simulink model "Nerthus_sim"  (R2021a)
settings: Solver=ode45  StartTime=0.0  StopTime=simtime  MaxStep=ts_max
values from neighbouring files (symbols this model uses):
  a_f = 1E-5*depl_fuel_temp_coef(depl_index)    [parameters.m]
  a_g = 1E-5*depl_grap_temp_coef(depl_index)    [parameters.m]
  A_s = 1.2245    [parameters.m]
  beta = depl_beta(depl_index,:)    [parameters.m]
  beta_t = sum(beta)    [parameters.m]
  Cp_1 = mean(interp1(Cal_temp1, Cal_Cp1, region_fdw))/1e3    [parameters.m]
  Cp_2 = mean(interp1(Cal_temp2, Cal_Cp2, region_sc))/1e3    [parameters.m]
  Cp_3 = mean(interp1(Cal_temp3, Cal_Cp3, region_s2))/1e3    [parameters.m]
  Cp_4 = mean(interp1(Cal_temp4, Cal_Cp4, region_s1))/1e3    [parameters.m]
  Cp_p = 0.00154912    [parameters.m]
  Cp_w = 456.056e-6    (= 0.000456056)    [parameters.m]
  D_it = 0.0141478    [parameters.m]
  D_ot = 0.015875    [parameters.m]
  DHRS_MODE = 1    [parameters.m]    (also in transients.m)
  DHRS_Power = P*(0.10)    (= 55.7)    [parameters.m]    (also in transients.m)
  DHRS_time = 20000000    [parameters.m]    (also in transients.m)
  DHRS_TIME_K = 10    [parameters.m]
  dHs_dPs = -0.042433622114357    (= -0.0424336221144)    [parameters.m]
  Epsilon = 1E-3    (= 0.001)    [parameters.m]
  Fiss_factor = 2.464783802008740e-03    (= 0.00246478380201)    [parameters.m]
  gamma0 = 9.635981959409105e-01    (= 0.963598195941)    [parameters.m]
  gamma1 = 3.560674858154914e-02    (= 0.0356067485815)    [parameters.m]
  gamma2 = 7.950554775404400e-04    (= 0.00079505547754)    [parameters.m]
  gamma_I = 5.1135e-2    (= 0.051135)    [parameters.m]
  gamma_Te = 6.1e-2    (= 0.061)    [parameters.m]
  gamma_Xe = 1.1628e-2    (= 0.011628)    [parameters.m]
  h_pw = h_s_shx    (= 0.00910134357894)    [parameters.m]
  H_s_table = zeros(m, n)    [parameters.m]
  h_wb = 13349.334646671E-6    (= 0.0133493346467)    [parameters.m]
  h_ws = 5732.378387768E-6    (= 0.00573237838777)    [parameters.m]
  h_wsc = 8385.005556375E-6    (= 0.00838500555638)    [parameters.m]
  hA_fg = 12.5325*SF_area_CORE    (= 12.5325)    [parameters.m]
  hA_p_phx1 = [UA_phx_nm,UA_phx_nm,UA_phx_nm,UA_phx_nm]    [parameters.m]
  hA_p_shx1 = [UA_shx_nm,UA_shx_nm,UA_shx_nm,UA_shx_nm]    [parameters.m]
  hA_s_phx1 = [UA_phx_nm,UA_phx_nm,UA_phx_nm,UA_phx_nm]    [parameters.m]
  hA_s_shx1 = [UA_shx_nm,UA_shx_nm,UA_shx_nm,UA_shx_nm]    [parameters.m]
  I_0 = ((gamma_I*Sig_f_msdr*phi_0) + (lam_Te*Te_0))/lam_I    (= 7.13664200441e+16)    [parameters.m]
  k_1 = 0.5    [parameters.m]
  K_1 = 11.632248097704855    (= 11.6322480977)    [parameters.m]
  k_2 = 0.5    [parameters.m]
  K_4 = b(1)    [parameters.m]
  K_5 = a(1)    [parameters.m]
  K_b = 12.834854076292217    (= 12.8348540763)    [parameters.m]
  k_f1 = k_f/nn_f    (= 0.465)    [parameters.m]
  k_f2 = k_f/nn_f    (= 0.465)    [parameters.m]
  k_g = 0.07    [parameters.m]
  K_pump = 10000000    [parameters.m]
  K_sc = -17.615718797133468    (= -17.6157187971)    [parameters.m]
  L = 8.5344*SF_length    (= 7.72866182253)    [parameters.m]
  L_b = 2.3645*SF_length    (= 2.14126603855)    [parameters.m]
  L_s = 4.723*SF_length    (= 4.27709854094)    [parameters.m]
  L_sc = 1.4469*SF_length    (= 1.31029724304)    [parameters.m]
  Lam = depl_Lam(depl_index)    [parameters.m]
  lam = [1.240E-02, 3.05E-02, 1.11E-01, 3.01E-01, 1.140E+00, 3.014E+00]    [parameters.m]
  lam_bubl = 2E-2    (= 0.02)    [parameters.m]
  lam_I = 2.875e-5    (= 2.875e-05)    [parameters.m]
  lam_Te = 3.65e-02    (= 0.0365)    [parameters.m]
  lam_Xe = 2.0916e-5    (= 2.0916e-05)    [parameters.m]
  lambda0 = 0.0945298    [parameters.m]
  lambda1 = 0.00441957    [parameters.m]
  lambda2 = 8.60979e-05    [parameters.m]
  m_f_t = mdot_fuel*(tau_core + tau_phx + tau_DHRS)    (= 116168.4)    [parameters.m]
  M_initial = L_b*rho_b*A_s + L_s*rho_s*A_s + L_sc*A_s*rho_sc    [parameters.m]
  M_stm = 0.018    [parameters.m]
  mcp_f1 = mn_f*scp_fuel    (= 62.07748875)    [parameters.m]
  mcp_f2 = mn_f*scp_fuel    (= 62.07748875)    [parameters.m]
  mcp_g1 = m_g*scp_graphite    (= 3731.2785)    [parameters.m]
  mcp_p_phx1 = scp_fuel*mp_phx1    [parameters.m]
  mcp_p_shx1 = scp_coolant*mp_shx1    [parameters.m]
  mcp_s_phx1 = scp_coolant*ms_phx1    [parameters.m]
  mcp_s_shx1 = scp_HITEC*ms_shx1    [parameters.m]
  mcp_t_phx1 = scp_tube*mt_phx1    [parameters.m]
  mcp_t_shx1 = scp_tube*mt_shx1    [parameters.m]
  mdot_coolant = 1543 + SF_fdw_PHX    (= 1543)    [parameters.m]
  mdot_HITEC = 3379 + SF_fdw_SHX    (= 3379)    [parameters.m]
  mn_f = (m_f/nn_f)    (= 31567.5)    [parameters.m]
  mn_piDHRS = mdot_fuel*tau_DHRS    (= 4209)    [parameters.m]
  mn_UHX = (tau_HITEC_UHX*mdot_HITEC)/n_UHX    (= 11263.3333333)    [parameters.m]
  mp_phx1 = [mp_phx_nm, mp_phx_nm, mp_phx_nm, mp_phx_nm]    [parameters.m]
  mp_shx1 = [mp_shx_nm, mp_shx_nm, mp_shx_nm, mp_shx_nm]    [parameters.m]
  ms_phx1 = [ms_phx_nm, ms_phx_nm, ms_phx_nm, ms_phx_nm]    [parameters.m]
  ms_shx1 = [ms_shx_nm, ms_shx_nm, ms_shx_nm, ms_shx_nm]    [parameters.m]
  N = 6546*SF_linear    (= 4861.496)    [parameters.m]
  n_frac0 = 1    [parameters.m]
  n_UHX = 3    [parameters.m]
  omega = 10.00000    (= 10)    [parameters.m]    (also in transients.m)
  P = 557    [parameters.m]    (also in transients.m)
  P_s = 12.5    [parameters.m]
  P_sat = 12.5    [parameters.m]
  P_sc = 12.5    [parameters.m]
  phi_0 = P/(3.04414e-17*1e6*Sig_f_msdr)    (= 3.1277117014e+14)    [parameters.m]
  Power_Bleed = P*(0.00)    (= 0)    [parameters.m]    (also in transients.m)
  pres_table = pres_inp    [parameters.m]
  R = 8.314462E-6    (= 8.314462e-06)    [parameters.m]
  rho_0 = beta_t - bterm    [parameters.m]
  rho_b = (XSteam('rho_pT', 125, 327.81) + XSteam('rho_pT', 125, 327.82))/2    [parameters.m]
  rho_p = rho_HITEC    (= 1680)    [parameters.m]
  rho_s = mean(interp1(Cal_temp_steam, Cal_rho3, region_steam))    [parameters.m]
  rho_sc = mean(interp1(Cal_temp2, Cal_rho2, region_sc))    [parameters.m]
  rho_w = 8425.712    [parameters.m]
  rhoXe_0 = (-sig_Xe / Sig_a) * (gamma_Te + gamma_I + gamma_Xe) * Sig_f_msdr * phi_0/(lam_Xe + sig_Xe * phi_0 + lam_bubl)    (= -0.000282704956487)    [parameters.m]
  scp_coolant = 8.83E-3    (= 0.00883)    [parameters.m]
  scp_fuel = 1.9665E-3    (= 0.0019665)    [parameters.m]
  scp_HITEC = 0.00154912    [parameters.m]
  Sig_f_msdr = U_den*U_sig    (= 0.058501076601)    [parameters.m]
  sig_Xe = 2.66449e-18    [parameters.m]
  sin_mag = 0    [parameters.m]    (also in transients.m)
  T0_f1 = Tf_in + (T0_f2-Tf_in)/2    (= 649.2)    [parameters.m]
  T0_f2 = 681.8    [parameters.m]
  T0_g1 = T0_f1 + (k_g*P/hA_fg)    (= 652.311111111)    [parameters.m]
  T0_p_phx1 = [663.1, 644.3, 630.3, 616.6]    [parameters.m]
  T0_p_shx1 = [641.8, 656.3, 621.4, 586.4]    [parameters.m]
  T0_s_phx1 = [595.1, 603.8, 615.6, 627.3]    [parameters.m]
  T0_s_shx1 = [598.2, 689.1, 651.4, 613.7]    [parameters.m]
  T0_t_phx1 = [639.3, 612.7]    [parameters.m]
  T0_t_shx1 = [646.6, 609.8]    [parameters.m]
  T_fw = 180.0    (= 180)    [parameters.m]
  T_p1 = 605.5    [parameters.m]
  T_p2 = 579.6    [parameters.m]
  T_p3 = 557.5    [parameters.m]
  ... (+40 more)
undefined symbols (not defined in the file or in its folder): C0, Cp_s, Cp_sc, ln, rho_f, scp_f, scp_s, vdot_f, vdot_s
libraries: pid_lib x1, simulink x1
(part 2 of 3)

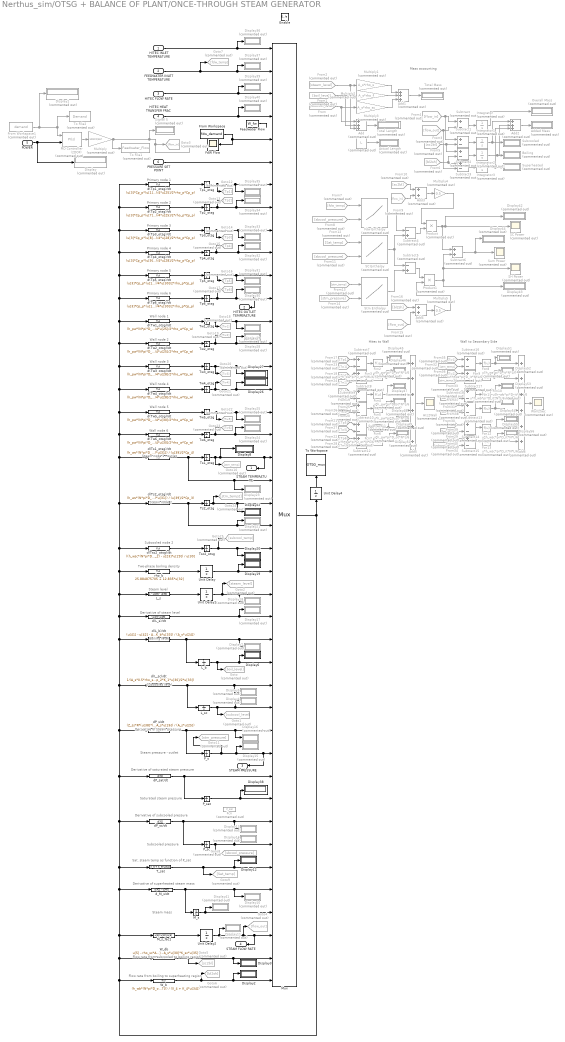
== system Nerthus_sim/OTSG + BALANCE OF PLANT/ONCE-THROUGH STEAM GENERATOR ==
  note: Wall to Secondary Side
  note: Hitec to Wall
  note: Mass accounting
  note: Primary node 1
  note: Primary node 2
  note: Primary node 3
  note: Primary node 4
  note: Primary node 5
  note: Primary node 6
  note: Wall node 1
  note: Wall node 2
  note: Wall node 3
  note: Wall node 4
  note: Wall node 5
  note: Wall node 6
  note: Steam node 1 - outlet
  note: Steam level
  note: Boiling level
  note: Subcooled level
  note: Derivative of saturated steam pressure
  note: Sat. steam temp as function of P_sat
  note: Saturated steam pressure
  note: Subcooled pressure
  note: Derivative of steam pressure
  note: Derivative of subcooled pressure
  note: Steam pressure - outlet
  note: Subcooled node 2
  note: Steam node 2
  note: Two-phase boiling density
  note: Derivative of superheated steam mass
  note: Steam mass
  note: Flow rate from subcooled to boiling region
  note: Flow rate from boiling to superheating region
  note: Derivative of steam level
  HITEC INLET TEMPERATURE : Inport
  FEEDWATER INLET TEMPERATURE : Inport  Port=2
  HITEC FLOW RATE : Inport  Port=3
  HITEC HEAT TRANSFER FRAC : Inport  Port=4
  POWER : Inport  Port=5
  PRESSURE SET POINT : Inport  Port=6
  Enable : EnablePort
  " " : Constant  Commented=on  Value=L
  "Actual Length " : Display  Commented=on
  Add : Sum  Commented=on  Inputs=+++
  Add1 : Sum  Commented=on  Inputs=+++
  Add2 : Sum  Commented=on  Inputs=+++
  Add3 : Sum  Commented=on
  Add4 : Sum  Commented=on
  Add5 : Sum  Commented=on  Inputs=++++++
  Add6 : Sum  Commented=on  Inputs=++++++
  Added Mass : Display  Commented=on
  Boiling : Display  Commented=on
  Display{,1,4..5,7,10..11,13..18,21,23..25,28..37,39..56} (45 alike) : Display  Commented=on
  Display{2..3,6,8,12,19..20,22,26..27,38} (11 alike) : Display
  Fcn : Fcn  Commented=on  Expr=P_sat
  Fcn10 : Fcn  Commented=on  Expr=u*h_wb*pi*D_it*N*L/6
  Fcn11 : Fcn  Commented=on  Expr=u*h_wb*pi*D_it*N*L/6
  Fcn12 : Fcn  Commented=on  Expr=u*h_wsc*pi*D_it*N*L/6
  Fcn13 : Fcn  Commented=on  Expr=u*h_wsc*pi*D_it*N*L/6
  Fcn{2..7} (6 alike) : Fcn  Commented=on  Expr=u*h_pw*pi*D_ot*N*L/6
  Fcn8 : Fcn  Commented=on  Expr=u*h_ws*pi*D_it*N*L/6
  Fcn9 : Fcn  Commented=on  Expr=u*h_ws*pi*D_it*N*L/6
  FdW Flow : Scope
  Fdw Enthalpy : Lookup_n-D  Commented=on  BreakpointsForDimension1=temp_table  BreakpointsForDimension2=pres_table  Table=H_s_table  DiagnosticForOutOfRangeInput=Warning  InternalRulePriority=Speed  RndMeth=Simplest  InputSameDT=on
      settings: InputPortMap=u0,u1
  Feedwater Flow : Constant  Value=W_fw
  From : From  Commented=on  GotoTag=subcool_level
  From Workspace : FromWorkspace  VariableName=fdw_demand
  From Workspace1 : FromWorkspace  Commented=on  VariableName=demand  SampleTime=1  Interpolate=off  OutputAfterFinalValue=Holding final value
  From1 : From  Commented=on  GotoTag=boil_level
  From10 : From  Commented=on  GotoTag=sc2bl
  From11 : From  Commented=on  GotoTag=sbcool_pressure
  From{12,29..31} (4 alike) : From  Commented=on  GotoTag=Sat_temp
  From13 : From  Commented=on  GotoTag=stm_temp
  From14 : From  Commented=on  GotoTag=stm_pressure
  From15 : From  Commented=on  GotoTag=flow_out
  From16 : From  Commented=on  GotoTag=bl2sh
  From17 : From  Commented=on  GotoTag=Tp1
  From18 : From  Commented=on  GotoTag=Tp2
  From19 : From  Commented=on  GotoTag=Tp3
  From2 : From  Commented=on  GotoTag=steam_level
  From20 : From  Commented=on  GotoTag=Tp4
  From21 : From  Commented=on  GotoTag=Tp5
  From22 : From  Commented=on  GotoTag=Tp6
  From23 : From  Commented=on  GotoTag=Tw1
  From24 : From  Commented=on  GotoTag=Tw2
  From25 : From  Commented=on  GotoTag=Tw3
  From26 : From  Commented=on  GotoTag=Tw4
  From27 : From  Commented=on  GotoTag=Tw5
  From28 : From  Commented=on  GotoTag=Tw6
  From3 : From  Commented=on  GotoTag=flow_out
  From32 : From  Commented=on  GotoTag=stm_temp
  From33 : From  Commented=on  GotoTag=stm_temp2
  From34 : From  Commented=on  GotoTag=subcool_temp
  From35 : From  Commented=on  GotoTag=Tw1
  From36 : From  Commented=on  GotoTag=Tw2
  From37 : From  Commented=on  GotoTag=Tw3
  From38 : From  Commented=on  GotoTag=Tw4
  From39 : From  Commented=on  GotoTag=Tw5
  From4 : From  Commented=on  GotoTag=flow_in
  From40 : From  Commented=on  GotoTag=Tw6
  From5 : From  Commented=on  GotoTag=sc2bl
  From6 : From  Commented=on  GotoTag=bl2sh
  From7 : From  Commented=on  GotoTag=fdw_temp
  From8 : From  Commented=on  GotoTag=sbcool_pressure
  From9 : From  Commented=on  GotoTag=flow_in
  Goto : Goto  Commented=on  GotoTag=boil_level
  Goto1 : Goto  Commented=on  GotoTag=subcool_level
  Goto10 : Goto  Commented=on  GotoTag=stm_temp
  Goto11 : Goto  Commented=on  GotoTag=stm_pressure
  Goto12 : Goto  Commented=on  GotoTag=Tp1
  Goto13 : Goto  Commented=on  GotoTag=Tp2
  Goto14 : Goto  Commented=on  GotoTag=Tp3
  Goto15 : Goto  Commented=on  GotoTag=Tp4
  Goto16 : Goto  Commented=on  GotoTag=Tp5
  Goto17 : Goto  Commented=on  GotoTag=Tp6
  Goto18 : Goto  Commented=on  GotoTag=Tw1
  Goto19 : Goto  Commented=on  GotoTag=Tw2
  Goto2 : Goto  Commented=on  GotoTag=steam_level
  Goto20 : Goto  Commented=on  GotoTag=Tw3
  Goto21 : Goto  Commented=on  GotoTag=Tw4
  Goto22 : Goto  Commented=on  GotoTag=Tw5
  Goto23 : Goto  Commented=on  GotoTag=Tw6
  Goto24 : Goto  Commented=on  GotoTag=stm_temp2
  Goto25 : Goto  Commented=on  GotoTag=subcool_temp
  Goto3 : Goto  Commented=on  GotoTag=flow_in
  Goto4 : Goto  Commented=on  GotoTag=flow_out
  Goto5 : Goto  Commented=on  GotoTag=sc2bl
  Goto6 : Goto  Commented=on  GotoTag=bl2sh
  Goto7 : Goto  Commented=on  GotoTag=fdw_temp
  Goto8 : Goto  Commented=on  GotoTag=sbcool_pressure
  Goto9 : Goto  Commented=on  GotoTag=Sat_temp
  Htc2Wall : Scope  Commented=on
  Integrator : Integrator  Commented=on  InitialCondition=M_initial
  Integrator1 : Integrator  Commented=on  InitialCondition=A_s*rho_sc*L_sc
  Integrator2 : Integrator  Commented=on  InitialCondition=A_s*rho_b*L_b
  Integrator3 : Integrator  Commented=on  InitialCondition=A_s*rho_s*L_s
  L_b : Integrator  InitialCondition=L_b  LimitOutput=on  LowerSaturationLimit=0.01
  L_s : Fcn  Expr=L - u[28] - u[30]
  L_sc : Integrator  InitialCondition=L_sc  LimitOutput=on  LowerSaturationLimit=0.01
  M_s : Integrator  InitialCondition=A_s*rho_s*L_s  LimitOutput=on  LowerSaturationLimit=1
  M_s_fac1 : Fcn  Expr=u[5]*u[32]/u[6]
  Multiply : Gain  Commented=on  Gain=1000*P/557
  Multiply1 : Gain  Commented=on  Gain=A_s*rho_s
  Multiply2 : Gain  Commented=on  Gain=A_s*rho_f
  Multiply3 : Gain  Commented=on  Gain=A_s*rho_sc
  Multiply4 : Gain  Commented=on  Gain=0.5
  Multiply5 : Gain  Commented=on  Gain=0.5
  Mux : Mux  Inputs=42
      settings: DisplayOption=signals
  Overall Mass : Display  Commented=on
  PID Controller (2DOF) : pid_lib/PID Controller (2DOF)  Commented=on  Controller=PI  Form=Parallel  TimeDomain=Continuous-time  UseExternalTs=off  SampleTime=-1  IntegratorMethod=Forward Euler  FilterMethod=Forward Euler  ControllerParametersSource=internal  P=0.003  I=0.001  D=-0.1  UseFilter=on  N=0.07  b=60  c=0.000385  TunerSelectOption=Transfer Function Based (PID Tuner App)  InitialConditionSource=internal  InitialConditionForIntegrator=0  InitialConditionForFilter=0  DifferentiatorICPrevScaledInput=0  ExternalReset=none  TrackingMode=off  Kt=1  LimitOutput=on  SatLimitsSource=internal  UpperSaturationLimit=2  LowerSaturationLimit=0.009  LinearizeAsGain=on  AntiWindupMode=none  Kb=1  POutMin=[]  POutMax=[]  IOutMin=[]  IOutMax=[]  DOutMin=[]  DOutMax=[]  NOutMin=[]  NOutMax=[]  bOutMin=[]  bOutMax=[]  cOutMin=[]  cOutMax=[]  SumOutMin=[]  SumOutMax=[]  SaturationOutMin=[]  SaturationOutMax=[]  PParamMin=[]  PParamMax=[]  IParamMin=[]  IParamMax=[]  DParamMin=[]  DParamMax=[]  NParamMin=[]  NParamMax=[]  bParamMin=[]  bParamMax=[]  cParamMin=[]  cParamMax=[]  KbParamMin=[]  KbParamMax=[]  KtParamMin=[]  KtParamMax=[]  KbOutMin=[]  KbOutMax=[]  KtOutMin=[]  KtOutMax=[]  IntegratorOutMin=[]  IntegratorOutMax=[]  FilterOutMin=[]  FilterOutMax=[]  SumI1OutMin=[]  SumI1OutMax=[]  SumI2OutMin=[]  SumI2OutMax=[]  SumI3OutMin=[]  SumI3OutMax=[]  SumI4OutMin=[]  SumI4OutMax=[]  SumDOutMin=[]  SumDOutMax=[]  Sum1OutMin=[]  Sum1OutMax=[]  Sum2OutMin=[]  Sum2OutMax=[]  Sum3OutMin=[]  Sum3OutMax=[]  DifferentiatorOutMin=[]  DifferentiatorOutMax=[]  FilterDiffOutCoefMin=[]  FilterDiffOutCoefMax=[]  ReciprocalOutMin=[]  ReciprocalOutMax=[]  SumDenOutMin=[]  SumDenOutMax=[]  SumNumOutMin=[]  SumNumOutMax=[]  DivideOutMin=[]  DivideOutMax=[]  UdiffTsProdOutMin=[]  UdiffTsProdOutMax=[]  NTsProdOutMin=[]  NTsProdOutMax=[]  UintegralTsProdOutMin=[]  UintegralTsProdOutMax=[]  UngainTsProdOutMin=[]  UngainTsProdOutMax=[]  IntegratorContinuousStateAttributes=''  IntegratorStateMustResolveToSignalObject=off  IntegratorRTWStateStorageClass=Auto  FilterContinuousStateAttributes=''  FilterStateMustResolveToSignalObject=off  FilterRTWStateStorageClass=Auto  ParallelPVariant=InternalParameters  IdealPVariant=Disabled  IVariant=InternalParameters  DVariant=Disabled  bVariant=InternalParameters  cVariant=Disabled  IntegratorVariant=Continuous  SatVariant=Enabled  AWVariant=Passthrough  PCopyVariant=Disabled  TRVariant=Disabled  FdbkBlocksVariant=Forward  IdealPFdbkVariant=Disabled  SatFdbkVariant=Disabled  DerivativeFilterVariant=Disabled  NVariant=Disabled  NCopyVariant=Disabled_SignalSpec  FilterICVariant=Disabled  IntegratorICVariant=InternalICs  ExternalResetVariant=Disabled  TRSumVariant=Passthrough  SumFdbkVariant=Disabled  SumVariant=Sum_PI  TsampFilterVariant=InternalTs  TsampNgainVariant=Passthrough  TsampIntegralVariant=Passthrough  ExternalSaturationOutDataTypeStr=Inherit: Same as second input
      settings: SourceProductBaseCode=SL
  P_s : Integrator  InitialCondition=P_s
  P_sat : Integrator  InitialCondition=P_sat
  P_sc : Integrator  InitialCondition=P_sc
  Product : Product  Commented=on
  Product1 : Product  Commented=on
  SC Enthalpy : Lookup_n-D  Commented=on  BreakpointsForDimension1=temp_table  BreakpointsForDimension2=pres_table  Table=H_s_table  DiagnosticForOutOfRangeInput=Warning  InternalRulePriority=Speed  RndMeth=Simplest  InputSameDT=on
      settings: InputPortMap=u0,u1
  SC Power : Scope  Commented=on
  SH Power : Scope  Commented=on
  Signal 5 : Display  Commented=on
  Stm Enthalpy : Lookup_n-D  Commented=on  BreakpointsForDimension1=temp_table  BreakpointsForDimension2=pres_table  Table=H_s_table  DiagnosticForOutOfRangeInput=Warning  InternalRulePriority=Speed  RndMeth=Simplest  InputSameDT=on
      settings: InputPortMap=u0,u1
  Subcooled : Display  Commented=on
  Subtract{,1..3,7..18} (16 alike) : Sum  Commented=on  Inputs=+-
  Subtract4 : Sum  Commented=on  Inputs=-+
  Subtract5 : Sum  Commented=on  Inputs=-+
  Subtract6 : Sum  Commented=on
  Sum Power : Scope  Commented=on
  Superheated : Display  Commented=on
  T_sat : Fcn  Expr=X_5 + K_5*u[34]
  To File1 : ToFile  Commented=on  Filename=Feedwater_Flow  MatrixName=Feedwater_Flow
  To File2 : ToFile  Commented=on  Filename=Demand  MatrixName=Demand
  To Workspace : ToWorkspace  VariableName=OTSG_mux  SaveFormat=Timeseries  SampleTime=-1
  Total Length : Display  Commented=on
  Total Mass : Display  Commented=on
  Tp1_otsg : Integrator  InitialCondition=T_p1
  Tp2_otsg : Integrator  InitialCondition=T_p2
  Tp3_otsg : Integrator  InitialCondition=T_p3
  Tp4_otsg : Integrator  InitialCondition=T_p4
  Tp5_otsg : Integrator  InitialCondition=T_p5
  Tp6_otsg : Integrator  InitialCondition=T_p6
  Ts1_otsg : Integrator  InitialCondition=T_s1
  Ts2_otsg : Integrator  InitialCondition=T_s2
  Tsc2_otsg : Integrator  InitialCondition=T_sc2
  Tw1_otsg : Integrator  InitialCondition=T_w1
  Tw2_otsg : Integrator  InitialCondition=T_w2
  Tw3_otsg : Integrator  InitialCondition=T_w3
  Tw4_otsg : Integrator  InitialCondition=T_w4
  Tw5_otsg : Integrator  InitialCondition=T_w5
  Tw6_otsg : Integrator  InitialCondition=T_w6
  Unit Delay : UnitDelay  InitialCondition=rho_b  SampleTime=-1  HasFrameUpgradeWarning=on
  Unit Delay1 : UnitDelay  InitialCondition=L_s  SampleTime=-1  HasFrameUpgradeWarning=on
  Unit Delay2 : UnitDelay  InitialCondition=W_fw  SampleTime=-1  HasFrameUpgradeWarning=on
  Unit Delay4 : UnitDelay  SampleTime=-1  HasFrameUpgradeWarning=on
  W_b : Fcn  Expr=(h_wb*(N*pi*D_ot*u[28])*(0.5*u[15] + 0.5*u[16] - u[37])) / (X_4 + K_4*u[34])
  W_db : Fcn  Expr=u[5] - rho_sc*A_s*u[29] - A_s*u[30]*K_sc*u[35]
  Wall2Sec : Scope  Commented=on
  d(L_b)/dt : Fcn  Expr=(u[41] - u[42] - A_s*u[28]*K_b*u[33]) / (A_s*u[24])
  d(L_s)/dt : Fcn  Expr=-u[27]-u[29]
  d(L_sc)/dt : Fcn  Expr=1/(A_s*0.5*rho_sc*Cp_2*(u[23] - u[37])) * (h_wsc*N*pi*D_ot*u[30]/2*(u[17] - u[37]) + Cp_2*(u[5]*u[23] - (u[5] + u[41])*0.5*u[37]) - A_s*u[30]/2*(K_sc*Cp_2*(u[23] - 2*u[37]) - 1)*u[35] - A_s*rho_sc*Cp_2*K_1*u[30]/2*u[33])
  d(Tp1_otsg)/dt : Fcn  Expr=(u[3]*Cp_p*(u[1] - u[7]) + h_pw*(N*pi*D_it*u[25]/2)*(u[13] - u[7])) / (N*pi*(D_it^2)/4*u[25]/2*rho_p*Cp_p)
  d(Tp2_otsg)/dt : Fcn  Expr=(u[3]*Cp_p*(u[7] - u[8]) + h_pw*(N*pi*D_it*u[25]/2)*(u[14] - u[8])) / (N*pi*(D_it^2)/4*u[25]/2*rho_p*Cp_p)
  d(Tp3_otsg)/dt : Fcn  Expr=(u[3]*Cp_p*(u[8] - u[9]) + h_pw*(N*pi*D_it*u[28]/2)*(u[15] - u[9])) / (N*pi*(D_it^2)/4*u[28]/2*rho_p*Cp_p)
  d(Tp4_otsg)/dt : Fcn  Expr=(u[3]*Cp_p*(u[9] - u[10]) + h_pw*(N*pi*D_it*u[28]/2)*(u[16] - u[10])) / (N*pi*(D_it^2)/4*u[28]/2*rho_p*Cp_p)
  d(Tp5_otsg)/dt : Fcn  Expr=(u[3]*Cp_p*(u[10] - u[11]) + h_pw*(N*pi*D_it*u[30]/2)*(u[17] - u[11])) / (N*pi*(D_it^2)/4*u[30]/2*rho_p*Cp_p)
  d(Tp6_otsg)/dt : Fcn  Expr=(u[3]*Cp_p*(u[11] - u[12]) + h_pw*(N*pi*D_it*u[30]/2)*(u[18] - u[12])) / (N*pi*(D_it^2)/4*u[30]/2*rho_p*Cp_p)
  d(Ts1_otsg)/dt : Fcn  Expr=(h_ws*(N*pi*D_ot*u[25]/2)*(u[13] - u[19]) + u[40]*Cp_4*(u[21] - u[19]) + Cp_4*(u[21] - u[19])*u[38]/2 + (A_s*u[25]/2 - u[39]/2*dHs_dPs)*u[31]) / (u[39]/2*Cp_4)
  d(Ts2_otsg)/dt : Fcn  Expr=(h_ws*(N*pi*D_ot*u[25]/2)*(u[14] - u[21]) + u[42]*Cp_3*(u[37] - u[21]) + (A_s*u[25]/2 - u[39]/2*dHs_dPs)*u[31]) / (u[39]/2*Cp_3)
  d(Tsc2_otsg)/dt : Fcn  Expr=((h_wsc*(N*pi*D_ot*u[30]/2)*(u[18] - u[23]) + (Cp_1*u[5]*u[2]) - Cp_2*((u[5] + u[41])*0.5*u[23]) + A_s*u[30]/2*u[35]) * 2/(A_s*rho_sc*Cp_2) - u[23]*u[29]) / u[30]
  d(Tw1_otsg)/dt : Fcn  Expr=(h_pw*(N*pi*D_it*u[25]/2)*(u[7] - u[13]) + h_ws*(N*pi*D_ot*u[25]/2)*(u[19] - u[13])) / (N*pi*(D_ot^2 - D_it^2)/4*u[25]/2*rho_w*Cp_w)
  d(Tw2_otsg)/dt : Fcn  Expr=(h_pw*(N*pi*D_it*u[25]/2)*(u[8] - u[14]) + h_ws*(N*pi*D_ot*u[25]/2)*(u[21] - u[14])) / (N*pi*(D_ot^2 - D_it^2)/4*u[25]/2*rho_w*Cp_w)
  d(Tw3_otsg)/dt : Fcn  Expr=(h_pw*(N*pi*D_it*u[28]/2)*(u[9] - u[15]) + h_wb*(N*pi*D_ot*u[28]/2)*(u[37] - u[15])) / (N*pi*(D_ot^2 - D_it^2)/4*u[28]/2*rho_w*Cp_w)
  d(Tw4_otsg)/dt : Fcn  Expr=(h_pw*(N*pi*D_it*u[28]/2)*(u[10] - u[16]) + h_wb*(N*pi*D_ot*u[28]/2)*(u[37] - u[16])) / (N*pi*(D_ot^2 - D_it^2)/4*u[28]/2*rho_w*Cp_w)
  d(Tw5_otsg)/dt : Fcn  Expr=(h_pw*(N*pi*D_it*u[30]/2)*(u[11] - u[17]) + h_wsc*(N*pi*D_ot*u[30]/2)*(u[37] - u[17])) / (N*pi*(D_ot^2 - D_it^2)/4*u[30]/2*rho_w*Cp_w)
  d(Tw6_otsg)/dt : Fcn  Expr=(h_pw*(N*pi*D_it*u[30]/2)*(u[12] - u[18]) + h_wsc*(N*pi*D_ot*u[30]/2)*(u[23] - u[18])) / (N*pi*(D_ot^2 - D_it^2)/4*u[30]/2*rho_w*Cp_w)
  dP_s/dt : Fcn  Expr=(Z_ss*R*(u[38]*(u[19] + u[21]) + u[39]*(u[20] + u[22]))/(2*M_stm) - u[32]*A_s*u[26]) / (A_s*u[25])
  dP_sat/dt : Fcn  Expr=u[31]
  dP_sc/dt : Fcn  Expr=u[31]
  d_M_s/dt : Fcn  Expr=u[42] - u[40]
  rho_b : Fcn  Expr=25.884875705 + 12.835*u[32]
  STEAM TEMPERATURE : Outport  VectorParamsAs1DForOutWhenUnconnected=off
  HITEC OUTLET TEMPERATURE : Outport  Port=2  VectorParamsAs1DForOutWhenUnconnected=off
  STEAM PRESSURE : Outport  Port=3  VectorParamsAs1DForOutWhenUnconnected=off
  STEAM FLOW RATE : Outport  Port=4  VectorParamsAs1DForOutWhenUnconnected=off
  wires:
  d(Tp1_otsg)/dt/1 -> Tp1_otsg/1
  HITEC INLET TEMPERATURE/1 -> Display36/1, Mux/1
  HITEC FLOW RATE/1 -> Display39/1, Mux/3
  HITEC HEAT TRANSFER FRAC/1 -> Display40/1, Mux/4
  PRESSURE SET POINT/1 -> Mux/6
  Tp1_otsg/1 -> Goto12/1, Display35/1, Mux/7
  Tp2_otsg/1 -> Goto13/1, Display34/1, Mux/8
  d(Tp2_otsg)/dt/1 -> Tp2_otsg/1
  Tp3_otsg/1 -> Goto14/1, Display33/1, Mux/9
  d(Tp3_otsg)/dt/1 -> Tp3_otsg/1
  Tp4_otsg/1 -> Goto15/1, Display32/1, Mux/10
  d(Tp4_otsg)/dt/1 -> Tp4_otsg/1
  Tp5_otsg/1 -> Goto16/1, Display31/1, Mux/11
  d(Tp5_otsg)/dt/1 -> Tp5_otsg/1
  d(Tp6_otsg)/dt/1 -> Tp6_otsg/1
  Tp6_otsg/1 -> Goto17/1, Display30/1, HITEC OUTLET TEMPERATURE/1, Mux/12
  d(Tw1_otsg)/dt/1 -> Tw1_otsg/1
  d(Tw2_otsg)/dt/1 -> Tw2_otsg/1
  Tw3_otsg/1 -> Goto20/1, Display27/1, Mux/15
  d(Tw3_otsg)/dt/1 -> Tw3_otsg/1
  d(Tw4_otsg)/dt/1 -> Tw4_otsg/1
  Tw4_otsg/1 -> Goto21/1, Display26/1, Mux/16
  Tw5_otsg/1 -> Goto22/1, Display25/1, Mux/17
  d(Tw5_otsg)/dt/1 -> Tw5_otsg/1
  d(Tw6_otsg)/dt/1 -> Tw6_otsg/1
  Tw6_otsg/1 -> Goto23/1, Display24/1, Mux/18
  L_sc/1 -> Goto1/1, Display4/1, Mux/30
  L_s/1 -> Unit Delay1/1
  L_b/1 -> Goto/1, Display6/1, Mux/28
  P_sat/1 -> Display38/1, Mux/34
  Tsc2_otsg/1 -> Goto25/1, Display20/1, Mux/23
  d(Tsc2_otsg)/dt/1 -> Tsc2_otsg/1
  Ts2_otsg/1 -> Goto24/1, Display22/1, Mux/21
  rho_b/1 -> Unit Delay/1
  Unit Delay/1 -> Display19/1, Mux/24
  d(Ts1_otsg)/dt/1 -> Display23/1, Mux/20, Ts1_otsg/1
  d(Ts2_otsg)/dt/1 -> Display21/1, Mux/22, Ts2_otsg/1
  dP_s/dt/1 -> Display16/1, Mux/31, P_s/1
  d(L_b)/dt/1 -> Display7/1, Mux/27, L_b/1
  d(L_s)/dt/1 -> Display17/1, Mux/26
  d(L_sc)/dt/1 -> Display5/1, Mux/29, L_sc/1
  dP_sat/dt/1 -> Mux/33, P_sat/1
  dP_sc/dt/1 -> Display13/1, Mux/35, P_sc/1
  Unit Delay1/1 -> Goto2/1, Display18/1, Mux/25
  T_sat/1 -> Goto9/1, Display12/1, Mux/37
  M_s_fac1/1 -> Unit Delay2/1
  d_M_s/dt/1 -> Display10/1, Mux/38, M_s/1
  Unit Delay4/1 -> To Workspace/1
  Tw1_otsg/1 -> Goto18/1, Display29/1, Mux/13
  From Workspace1/1 -> PID Controller (2DOF)/1, To File2/1, Display1/1
  Ts1_otsg/1 -> Goto10/1, STEAM TEMPERATURE/1, Mux/19, Display8/1
  POWER/1 -> PID Controller (2DOF)/2, Display/1
  Tw2_otsg/1 -> Goto19/1, Display28/1, Mux/14
  P_s/1 -> Goto11/1, Display15/1, Mux/32, STEAM PRESSURE/1
  Unit Delay2/1 -> Goto4/1, STEAM FLOW RATE/1, Mux/40, Display11/1
  P_sc/1 -> Goto8/1, Display14/1, Mux/36
  FEEDWATER INLET TEMPERATURE/1 -> Goto7/1, Display37/1, Mux/2
  PID Controller (2DOF)/1 -> Multiply/1
  From/1 -> Add/1, Multiply3/1
  From1/1 -> Multiply2/1, Add/2
  From2/1 -> Add/3, Multiply1/1
  Add/1 -> Total Length/1
  " "/1 -> "Actual Length "/1
  Multiply3/1 -> Add1/3
  Multiply2/1 -> Add1/2
  Multiply1/1 -> Add1/1
  Add1/1 -> Total Mass/1
  From4/1 -> Subtract1/1, Subtract/1
  From3/1 -> Subtract3/2, Subtract/2
  Subtract/1 -> Integrator/1
  M_s/1 -> Display41/1, Mux/39
  From5/1 -> Subtract2/1, Subtract1/2
  Subtract1/1 -> Integrator1/1
  Integrator1/1 -> Add2/1, Subcooled/1
  From6/1 -> Subtract2/2, Subtract3/1
  Integrator2/1 -> Add2/2, Boiling/1
  Subtract2/1 -> Integrator2/1
  Integrator3/1 -> Add2/3, Superheated/1
  Subtract3/1 -> Integrator3/1
  Add2/1 -> Added Mass/1
  Integrator/1 -> Overall Mass/1
  From7/1 -> Fdw Enthalpy/1
  From8/1 -> Fdw Enthalpy/2
  Fdw Enthalpy/1 -> Subtract4/1
  From9/1 -> Add3/2
  Product/1 -> Subtract6/1, Display42/1, SC Power/1
  From10/1 -> Add3/1
  Add3/1 -> Multiply4/1
  From11/1 -> SC Enthalpy/2
  From12/1 -> SC Enthalpy/1
  SC Enthalpy/1 -> Subtract4/2, Subtract5/1
  Multiply4/1 -> Product/1
  Subtract4/1 -> Product/2
  Stm Enthalpy/1 -> Subtract5/2
  From13/1 -> Stm Enthalpy/1
  From14/1 -> Stm Enthalpy/2
  From16/1 -> Add4/1
  Add4/1 -> Multiply5/1
  Multiply5/1 -> Product1/2
  From15/1 -> Add4/2
  Subtract5/1 -> Product1/1
  Product1/1 -> Subtract6/2, SH Power/1, Display43/1
  Subtract6/1 -> Display44/1, Sum Power/1
  From17/1 -> Subtract7/1
  From23/1 -> Subtract7/2
  From18/1 -> Subtract8/1
  From24/1 -> Subtract8/2
  From19/1 -> Subtract9/1
  From25/1 -> Subtract9/2
  From26/1 -> Subtract10/2
  From20/1 -> Subtract10/1
  From21/1 -> Subtract11/1
  From27/1 -> Subtract11/2
  From22/1 -> Subtract12/1
  From28/1 -> Subtract12/2
  Subtract7/1 -> Fcn2/1
  Subtract8/1 -> Fcn3/1
  Subtract9/1 -> Fcn4/1
  Subtract10/1 -> Fcn5/1
  Subtract11/1 -> Fcn6/1
  Subtract12/1 -> Fcn7/1
  Fcn2/1 -> Display45/1, Add5/1
  Fcn3/1 -> Display46/1, Add5/2
  Fcn4/1 -> Display47/1, Add5/3
  Fcn5/1 -> Display48/1, Add5/4
  Fcn6/1 -> Display49/1, Add5/5
  Fcn7/1 -> Display50/1, Add5/6
  Add5/1 -> Htc2Wall/1
  Fcn9/1 -> Display52/1, Add6/2
  Add6/1 -> Wall2Sec/1
  Fcn10/1 -> Display53/1, Add6/3
  Fcn12/1 -> Display55/1, Add6/5
  Fcn13/1 -> Display56/1, Add6/6
  Fcn11/1 -> Display54/1, Add6/4
  Subtract16/1 -> Fcn8/1
  From36/1 -> Subtract17/1
  Fcn8/1 -> Display51/1, Add6/1
  Subtract13/1 -> Fcn11/1
  Subtract15/1 -> Fcn13/1
  From35/1 -> Subtract16/1
  Subtract17/1 -> Fcn9/1
  Subtract18/1 -> Fcn10/1
  Subtract14/1 -> Fcn12/1
  From40/1 -> Subtract15/1
  From39/1 -> Subtract14/1
  From37/1 -> Subtract18/1
  From38/1 -> Subtract13/1
  From29/1 -> Subtract14/2
  From30/1 -> Subtract13/2
  From31/1 -> Subtract18/2
  From32/1 -> Subtract16/2
  From33/1 -> Subtract17/2
  From34/1 -> Subtract15/2
  Multiply/1 -> To File1/1, Signal 5/1, Goto3/1
  Feedwater Flow/1 -> ?
  From Workspace/1 -> FdW Flow/1, Mux/5
  Mux/1 -> W_b/1, W_db/1, d_M_s/dt/1, T_sat/1, dP_sc/dt/1, dP_sat/dt/1, dP_s/dt/1, d(L_sc)/dt/1, d(L_b)/dt/1, d(L_s)/dt/1, L_s/1, rho_b/1, d(Tsc2_otsg)/dt/1, d(Ts2_otsg)/dt/1, d(Ts1_otsg)/dt/1, d(Tw6_otsg)/dt/1, d(Tw5_otsg)/dt/1, d(Tw4_otsg)/dt/1, d(Tw3_otsg)/dt/1, d(Tw2_otsg)/dt/1, d(Tw1_otsg)/dt/1, d(Tp6_otsg)/dt/1, d(Tp5_otsg)/dt/1, d(Tp4_otsg)/dt/1, d(Tp3_otsg)/dt/1, d(Tp2_otsg)/dt/1, d(Tp1_otsg)/dt/1, M_s_fac1/1, Unit Delay4/1
  W_b/1 -> Display2/1, Mux/42, Goto6/1
  W_db/1 -> Display3/1, Mux/41, Goto5/1

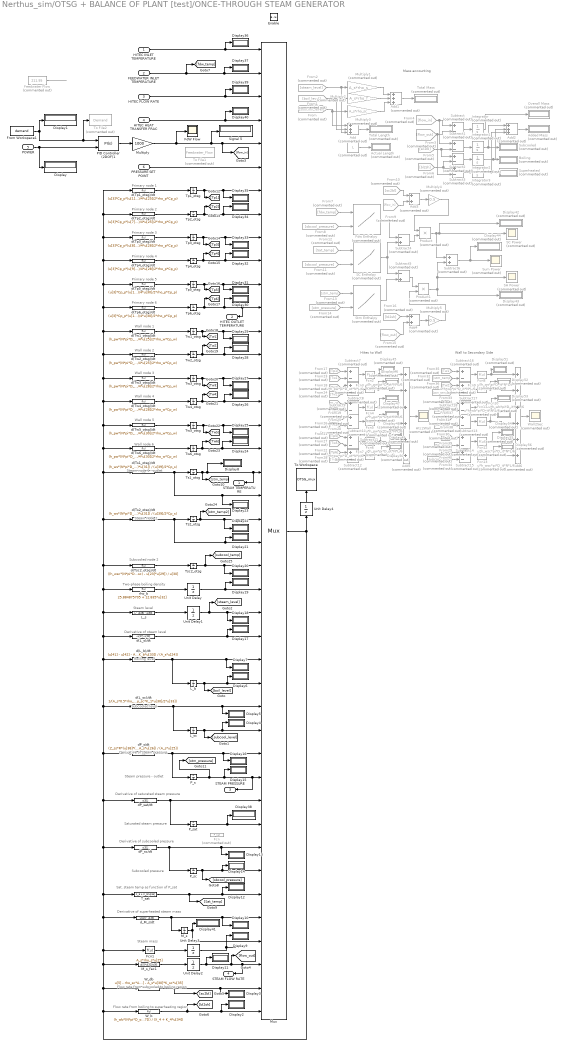
== system Nerthus_sim/OTSG + BALANCE OF PLANT [test]/ONCE-THROUGH STEAM GENERATOR ==
  note: Wall to Secondary Side
  note: Hitec to Wall
  note: Mass accounting
  note: Primary node 1
  note: Primary node 2
  note: Primary node 3
  note: Primary node 4
  note: Primary node 5
  note: Primary node 6
  note: Wall node 1
  note: Wall node 2
  note: Wall node 3
  note: Wall node 4
  note: Wall node 5
  note: Wall node 6
  note: Steam node 1 - outlet
  note: Steam level
  note: Boiling level
  note: Subcooled level
  note: Derivative of saturated steam pressure
  note: Sat. steam temp as function of P_sat
  note: Saturated steam pressure
  note: Subcooled pressure
  note: Derivative of steam pressure
  note: Derivative of subcooled pressure
  note: Steam pressure - outlet
  note: Subcooled node 2
  note: Steam node 2
  note: Two-phase boiling density
  note: Derivative of superheated steam mass
  note: Steam mass
  note: Flow rate from subcooled to boiling region
  note: Flow rate from boiling to superheating region
  note: Derivative of steam level
  HITEC INLET TEMPERATURE : Inport
  FEEDWATER INLET TEMPERATURE : Inport  Port=2
  HITEC FLOW RATE : Inport  Port=3
  HITEC HEAT TRANSFER FRAC : Inport  Port=4
  POWER : Inport  Port=5
  PRESSURE SET POINT : Inport  Port=6
  Enable : EnablePort
  " " : Constant  Commented=on  Value=L
  "Actual Length " : Display  Commented=on
  Add : Sum  Commented=on  Inputs=+++
  Add1 : Sum  Commented=on  Inputs=+++
  Add2 : Sum  Commented=on  Inputs=+++
  Add3 : Sum  Commented=on
  Add4 : Sum  Commented=on
  Add5 : Sum  Commented=on  Inputs=++++++
  Add6 : Sum  Commented=on  Inputs=++++++
  Added Mass : Display  Commented=on
  Boiling : Display  Commented=on
  Display{,1..41} (42 alike) : Display
  Display{42..56} (15 alike) : Display  Commented=on
  Fcn : Fcn  Commented=on  Expr=P_sat
  Fcn1 : Fcn  Expr=A_s*rho_s*u[25]
  Fcn10 : Fcn  Commented=on  Expr=u*h_wb*pi*D_it*N*L/6
  Fcn11 : Fcn  Commented=on  Expr=u*h_wb*pi*D_it*N*L/6
  Fcn12 : Fcn  Commented=on  Expr=u*h_wsc*pi*D_it*N*L/6
  Fcn13 : Fcn  Commented=on  Expr=u*h_wsc*pi*D_it*N*L/6
  Fcn{2..7} (6 alike) : Fcn  Commented=on  Expr=u*h_pw*pi*D_ot*N*L/6
  Fcn8 : Fcn  Commented=on  Expr=u*h_ws*pi*D_it*N*L/6
  Fcn9 : Fcn  Commented=on  Expr=u*h_ws*pi*D_it*N*L/6
  FdW Flow : Scope
  Fdw Enthalpy : Lookup_n-D  Commented=on  BreakpointsForDimension1=temp_table  BreakpointsForDimension2=pres_table  Table=H_s_table  DiagnosticForOutOfRangeInput=Warning  InternalRulePriority=Speed  RndMeth=Simplest  InputSameDT=on
      settings: InputPortMap=u0,u1
  "Feedwater Flow " : Constant  Commented=on  Value=211.95
  From : From  Commented=on  GotoTag=subcool_level
  From Workspace1 : FromWorkspace  VariableName=demand  SampleTime=1  Interpolate=off  OutputAfterFinalValue=Holding final value
  From1 : From  Commented=on  GotoTag=boil_level
  From10 : From  Commented=on  GotoTag=sc2bl
  From11 : From  Commented=on  GotoTag=sbcool_pressure
  From{12,29..31} (4 alike) : From  Commented=on  GotoTag=Sat_temp
  From13 : From  Commented=on  GotoTag=stm_temp
  From14 : From  Commented=on  GotoTag=stm_pressure
  From15 : From  Commented=on  GotoTag=flow_out
  From16 : From  Commented=on  GotoTag=bl2sh
  From17 : From  Commented=on  GotoTag=Tp1
  From18 : From  Commented=on  GotoTag=Tp2
  From19 : From  Commented=on  GotoTag=Tp3
  From2 : From  Commented=on  GotoTag=steam_level
  From20 : From  Commented=on  GotoTag=Tp4
  From21 : From  Commented=on  GotoTag=Tp5
  From22 : From  Commented=on  GotoTag=Tp6
  From23 : From  Commented=on  GotoTag=Tw1
  From24 : From  Commented=on  GotoTag=Tw2
  From25 : From  Commented=on  GotoTag=Tw3
  From26 : From  Commented=on  GotoTag=Tw4
  From27 : From  Commented=on  GotoTag=Tw5
  From28 : From  Commented=on  GotoTag=Tw6
  From3 : From  Commented=on  GotoTag=flow_out
  From32 : From  Commented=on  GotoTag=stm_temp
  From33 : From  Commented=on  GotoTag=stm_temp2
  From34 : From  Commented=on  GotoTag=subcool_temp
  From35 : From  Commented=on  GotoTag=Tw1
  From36 : From  Commented=on  GotoTag=Tw2
  From37 : From  Commented=on  GotoTag=Tw3
  From38 : From  Commented=on  GotoTag=Tw4
  From39 : From  Commented=on  GotoTag=Tw5
  From4 : From  Commented=on  GotoTag=flow_in
  From40 : From  Commented=on  GotoTag=Tw6
  From5 : From  Commented=on  GotoTag=sc2bl
  From6 : From  Commented=on  GotoTag=bl2sh
  From7 : From  Commented=on  GotoTag=fdw_temp
  From8 : From  Commented=on  GotoTag=sbcool_pressure
  From9 : From  Commented=on  GotoTag=flow_in
  Htc2Wall : Scope  Commented=on
  Integrator : Integrator  Commented=on  InitialCondition=M_initial
  Integrator1 : Integrator  Commented=on  InitialCondition=A_s*rho_sc*L_sc
  Integrator2 : Integrator  Commented=on  InitialCondition=A_s*rho_b*L_b
  Integrator3 : Integrator  Commented=on  InitialCondition=A_s*rho_s*L_s
  L_b : Integrator  InitialCondition=L_b
  L_s : Fcn  Expr=L - u[28] - u[30]
  L_sc : Integrator  InitialCondition=L_sc
  M_s : Integrator  InitialCondition=A_s*rho_s*L_s
  M_s_fac1 : Fcn  Expr=u[5]*u[32]/u[6]
  Multiply : Gain  Gain=1000
  Multiply1 : Gain  Commented=on  Gain=A_s*rho_s
  Multiply2 : Gain  Commented=on  Gain=A_s*rho_f
  Multiply3 : Gain  Commented=on  Gain=A_s*rho_sc
  Multiply4 : Gain  Commented=on  Gain=0.5
  Multiply5 : Gain  Commented=on  Gain=0.5
  Mux : Mux  Inputs=42
      settings: DisplayOption=signals
  Overall Mass : Display  Commented=on
  PID Controller (2DOF)1 : simulink/Continuous/PID Controller (2DOF)  Controller=PI  Form=Parallel  TimeDomain=Continuous-time  SampleTime=-1  IntegratorMethod=Forward Euler  FilterMethod=Forward Euler  ControllerParametersSource=internal  P=0.003  I=0.001  D=-0.1  UseFilter=on  N=0.07  b=60  c=0.000385  TunerSelectOption=Transfer Function Based (PID Tuner App)  InitialConditionSource=internal  InitialConditionForIntegrator=0  InitialConditionForFilter=0  DifferentiatorICPrevScaledInput=0  ExternalReset=none  TrackingMode=off  Kt=1  LimitOutput=on  UpperSaturationLimit=2  LowerSaturationLimit=0.001  LinearizeAsGain=on  AntiWindupMode=none  Kb=1  POutMin=[]  POutMax=[]  IOutMin=[]  IOutMax=[]  DOutMin=[]  DOutMax=[]  NOutMin=[]  NOutMax=[]  bOutMin=[]  bOutMax=[]  cOutMin=[]  cOutMax=[]  SumOutMin=[]  SumOutMax=[]  SaturationOutMin=[]  SaturationOutMax=[]  PParamMin=[]  PParamMax=[]  IParamMin=[]  IParamMax=[]  DParamMin=[]  DParamMax=[]  NParamMin=[]  NParamMax=[]  bParamMin=[]  bParamMax=[]  cParamMin=[]  cParamMax=[]  KbParamMin=[]  KbParamMax=[]  KtParamMin=[]  KtParamMax=[]  KbOutMin=[]  KbOutMax=[]  KtOutMin=[]  KtOutMax=[]  IntegratorOutMin=[]  IntegratorOutMax=[]  FilterOutMin=[]  FilterOutMax=[]  SumI1OutMin=[]  SumI1OutMax=[]  SumI2OutMin=[]  SumI2OutMax=[]  SumI3OutMin=[]  SumI3OutMax=[]  SumI4OutMin=[]  SumI4OutMax=[]  SumDOutMin=[]  SumDOutMax=[]  Sum1OutMin=[]  Sum1OutMax=[]  Sum2OutMin=[]  Sum2OutMax=[]  Sum3OutMin=[]  Sum3OutMax=[]  DifferentiatorOutMin=[]  DifferentiatorOutMax=[]  FilterDiffOutCoefMin=[]  FilterDiffOutCoefMax=[]  ReciprocalOutMin=[]  ReciprocalOutMax=[]  SumDenOutMin=[]  SumDenOutMax=[]  SumNumOutMin=[]  SumNumOutMax=[]  DivideOutMin=[]  DivideOutMax=[]  IntegratorContinuousStateAttributes=''  IntegratorStateMustResolveToSignalObject=off  IntegratorRTWStateStorageClass=Auto  FilterContinuousStateAttributes=''  FilterStateMustResolveToSignalObject=off  FilterRTWStateStorageClass=Auto  ParallelPVariant=InternalParameters  IdealPVariant=Disabled  IVariant=InternalParameters  DVariant=Disabled  bVariant=InternalParameters  cVariant=Disabled  IntegratorVariant=Continuous  SatVariant=Enabled  AWVariant=Passthrough  PCopyVariant=Disabled  TRVariant=Disabled  FdbkBlocksVariant=Forward  IdealPFdbkVariant=Disabled  SatFdbkVariant=Disabled  DerivativeFilterVariant=Disabled  NVariant=Disabled  NCopyVariant=Disabled_SignalSpec  FilterICVariant=Disabled  IntegratorICVariant=InternalICs  ExternalResetVariant=Disabled  TRSumVariant=Passthrough  SumFdbkVariant=Disabled  SumVariant=Sum_PI
  P_s : Integrator  InitialCondition=P_s
  P_sat : Integrator  InitialCondition=P_sat
  P_sc : Integrator  InitialCondition=P_sc
  Product : Product  Commented=on
  Product1 : Product  Commented=on
  SC Enthalpy : Lookup_n-D  Commented=on  BreakpointsForDimension1=temp_table  BreakpointsForDimension2=pres_table  Table=H_s_table  DiagnosticForOutOfRangeInput=Warning  InternalRulePriority=Speed  RndMeth=Simplest  InputSameDT=on
      settings: InputPortMap=u0,u1
  SC Power : Scope  Commented=on
  SH Power : Scope  Commented=on
  Signal 5 : Display
  Stm Enthalpy : Lookup_n-D  Commented=on  BreakpointsForDimension1=temp_table  BreakpointsForDimension2=pres_table  Table=H_s_table  DiagnosticForOutOfRangeInput=Warning  InternalRulePriority=Speed  RndMeth=Simplest  InputSameDT=on
      settings: InputPortMap=u0,u1
  Subcooled : Display  Commented=on
  Subtract{,1..3,7..18} (16 alike) : Sum  Commented=on  Inputs=+-
  Subtract4 : Sum  Commented=on  Inputs=-+
  Subtract5 : Sum  Commented=on  Inputs=-+
  Subtract6 : Sum  Commented=on
  Sum Power : Scope  Commented=on
  Superheated : Display  Commented=on
  T_sat : Fcn  Expr=X_5 + K_5*u[34]
  To File1 : ToFile  Commented=on  Filename=Feedwater_Flow  MatrixName=Feedwater_Flow
  To File2 : ToFile  Commented=on  Filename=Demand  MatrixName=Demand
  To Workspace : ToWorkspace  VariableName=OTSG_mux  SaveFormat=Timeseries  SampleTime=-1
  Total Length : Display  Commented=on
  Total Mass : Display  Commented=on
  Tp1_otsg : Integrator  InitialCondition=T_p1
  Tp2_otsg : Integrator  InitialCondition=T_p2
  Tp3_otsg : Integrator  InitialCondition=T_p3
  Tp4_otsg : Integrator  InitialCondition=T_p4
  Tp5_otsg : Integrator  InitialCondition=T_p5
  Tp6_otsg : Integrator  InitialCondition=T_p6
  Ts1_otsg : Integrator  InitialCondition=T_s1
  Ts2_otsg : Integrator  InitialCondition=T_s2
  Tsc2_otsg : Integrator  InitialCondition=T_sc2
  Tw1_otsg : Integrator  InitialCondition=T_w1
  Tw2_otsg : Integrator  InitialCondition=T_w2
  Tw3_otsg : Integrator  InitialCondition=T_w3
  Tw4_otsg : Integrator  InitialCondition=T_w4
  Tw5_otsg : Integrator  InitialCondition=T_w5
  Tw6_otsg : Integrator  InitialCondition=T_w6
  Unit Delay : UnitDelay  InitialCondition=rho_b  SampleTime=-1  HasFrameUpgradeWarning=on
  Unit Delay1 : UnitDelay  InitialCondition=L_s  SampleTime=-1  HasFrameUpgradeWarning=on
  Unit Delay2 : UnitDelay  InitialCondition=W_fw  SampleTime=-1  HasFrameUpgradeWarning=on
  Unit Delay3 : UnitDelay  InitialCondition=A_s*rho_s*L_s  SampleTime=-1  HasFrameUpgradeWarning=on
  Unit Delay4 : UnitDelay  SampleTime=-1  HasFrameUpgradeWarning=on
  W_b : Fcn  Expr=(h_wb*(N*pi*D_ot*u[28])*(0.5*u[15] + 0.5*u[16] - u[37])) / (X_4 + K_4*u[34])
  W_db : Fcn  Expr=u[5] - rho_sc*A_s*u[29] - A_s*u[30]*K_sc*u[35]
  Wall2Sec : Scope  Commented=on
  d(L_b)/dt : Fcn  Expr=(u[41] - u[42] - A_s*u[28]*K_b*u[33]) / (A_s*u[24])
  d(L_s)/dt : Fcn  Expr=-u[27]-u[29]
  d(L_sc)/dt : Fcn  Expr=1/(A_s*0.5*rho_sc*Cp_sc*(u[23] - u[37])) * (h_wsc*N*pi*D_ot*u[30]/2*(u[17] - u[37]) + Cp_sc*(u[5]*u[23] - (u[5] + u[41])*0.5*u[37]) - A_s*u[30]/2*(K_sc*Cp_sc*(u[23] - 2*u[37]) - 1)*u[35] - A_s*rho_sc*Cp_sc*K_1*u[30]/2*u[33])
  d(Tp1_otsg)/dt : Fcn  Expr=(u[3]*Cp_p*(u[1] - u[7]) + h_pw*(N*pi*D_it*u[25]/2)*(u[13] - u[7])) / (N*pi*(D_it^2)/4*u[25]/2*rho_p*Cp_p)
  d(Tp2_otsg)/dt : Fcn  Expr=(u[3]*Cp_p*(u[7] - u[8]) + h_pw*(N*pi*D_it*u[25]/2)*(u[14] - u[8])) / (N*pi*(D_it^2)/4*u[25]/2*rho_p*Cp_p)
  d(Tp3_otsg)/dt : Fcn  Expr=(u[3]*Cp_p*(u[8] - u[9]) + h_pw*(N*pi*D_it*u[28]/2)*(u[15] - u[9])) / (N*pi*(D_it^2)/4*u[28]/2*rho_p*Cp_p)
  d(Tp4_otsg)/dt : Fcn  Expr=(u[3]*Cp_p*(u[9] - u[10]) + h_pw*(N*pi*D_it*u[28]/2)*(u[16] - u[10])) / (N*pi*(D_it^2)/4*u[28]/2*rho_p*Cp_p)
  d(Tp5_otsg)/dt : Fcn  Expr=(u[3]*Cp_p*(u[10] - u[11]) + h_pw*(N*pi*D_it*u[30]/2)*(u[17] - u[11])) / (N*pi*(D_it^2)/4*u[30]/2*rho_p*Cp_p)
  d(Tp6_otsg)/dt : Fcn  Expr=(u[3]*Cp_p*(u[11] - u[12]) + h_pw*(N*pi*D_it*u[30]/2)*(u[18] - u[12])) / (N*pi*(D_it^2)/4*u[30]/2*rho_p*Cp_p)
  d(Ts1_otsg)/dt : Fcn  Expr=(h_ws*(N*pi*D_ot*u[25]/2)*(u[13] - u[19]) + u[40]*Cp_s*(u[21] - u[19]) + Cp_s*(u[21] - u[19])*u[38]/2 + (A_s*u[25]/2 - u[39]/2*dHs_dPs)*u[31]) / (u[39]/2*Cp_s)
  d(Ts2_otsg)/dt : Fcn  Expr=(h_ws*(N*pi*D_ot*u[25]/2)*(u[14] - u[21]) + u[42]*Cp_s*(u[37] - u[21]) + (A_s*u[25]/2 - u[39]/2*dHs_dPs)*u[31]) / (u[39]/2*Cp_s)
  d(Tsc2_otsg)/dt : Fcn  Expr=((h_wsc*(N*pi*D_ot*u[30]/2)*(u[18] - u[23]) + Cp_sc*(u[5]*u[2] - (u[5] + u[41])*0.5*u[23]) + A_s*u[30]/2*u[35]) * 2/(A_s*rho_sc*Cp_sc) - u[23]*u[29]) / u[30]
  d(Tw1_otsg)/dt : Fcn  Expr=(h_pw*(N*pi*D_it*u[25]/2)*(u[7] - u[13]) + h_ws*(N*pi*D_ot*u[25]/2)*(u[19] - u[13])) / (N*pi*(D_ot^2 - D_it^2)/4*u[25]/2*rho_w*Cp_w)
  d(Tw2_otsg)/dt : Fcn  Expr=(h_pw*(N*pi*D_it*u[25]/2)*(u[8] - u[14]) + h_ws*(N*pi*D_ot*u[25]/2)*(u[21] - u[14])) / (N*pi*(D_ot^2 - D_it^2)/4*u[25]/2*rho_w*Cp_w)
  d(Tw3_otsg)/dt : Fcn  Expr=(h_pw*(N*pi*D_it*u[28]/2)*(u[9] - u[15]) + h_wb*(N*pi*D_ot*u[28]/2)*(u[37] - u[15])) / (N*pi*(D_ot^2 - D_it^2)/4*u[28]/2*rho_w*Cp_w)
  d(Tw4_otsg)/dt : Fcn  Expr=(h_pw*(N*pi*D_it*u[28]/2)*(u[10] - u[16]) + h_wb*(N*pi*D_ot*u[28]/2)*(u[37] - u[16])) / (N*pi*(D_ot^2 - D_it^2)/4*u[28]/2*rho_w*Cp_w)
  d(Tw5_otsg)/dt : Fcn  Expr=(h_pw*(N*pi*D_it*u[30]/2)*(u[11] - u[17]) + h_wsc*(N*pi*D_ot*u[30]/2)*(u[37] - u[17])) / (N*pi*(D_ot^2 - D_it^2)/4*u[30]/2*rho_w*Cp_w)
  d(Tw6_otsg)/dt : Fcn  Expr=(h_pw*(N*pi*D_it*u[30]/2)*(u[12] - u[18]) + h_wsc*(N*pi*D_ot*u[30]/2)*(u[23] - u[18])) / (N*pi*(D_ot^2 - D_it^2)/4*u[30]/2*rho_w*Cp_w)
  dP_s/dt : Fcn  Expr=(Z_ss*R*(u[38]*(u[19] + u[21]) + u[39]*(u[20] + u[22]))/(2*M_stm) - u[32]*A_s*u[26]) / (A_s*u[25])
  dP_sat/dt : Fcn  Expr=u[31]
  dP_sc/dt : Fcn  Expr=u[31]
  d_M_s/dt : Fcn  Expr=u[42] - u[40]
  rho_b : Fcn  Expr=25.884875705 + 12.835*u[32]
  STEAM TEMPERATURE : Outport  VectorParamsAs1DForOutWhenUnconnected=off
  HITEC OUTLET TEMPERATURE : Outport  Port=2  VectorParamsAs1DForOutWhenUnconnected=off
  STEAM PRESSURE : Outport  Port=3  VectorParamsAs1DForOutWhenUnconnected=off
  STEAM FLOW RATE : Outport  Port=4  VectorParamsAs1DForOutWhenUnconnected=off
  wires:
  d(Tp1_otsg)/dt/1 -> Tp1_otsg/1
  HITEC INLET TEMPERATURE/1 -> Display36/1, Mux/1
  HITEC FLOW RATE/1 -> Display39/1, Mux/3
  HITEC HEAT TRANSFER FRAC/1 -> Display40/1, Mux/4
  PRESSURE SET POINT/1 -> Mux/6
  Tp1_otsg/1 -> [Tp1], Display35/1, Mux/7
  Tp2_otsg/1 -> [Tp2], Display34/1, Mux/8
  d(Tp2_otsg)/dt/1 -> Tp2_otsg/1
  Tp3_otsg/1 -> [Tp3], Display33/1, Mux/9
  d(Tp3_otsg)/dt/1 -> Tp3_otsg/1
  Tp4_otsg/1 -> [Tp4], Display32/1, Mux/10
  d(Tp4_otsg)/dt/1 -> Tp4_otsg/1
  Tp5_otsg/1 -> [Tp5], Display31/1, Mux/11
  d(Tp5_otsg)/dt/1 -> Tp5_otsg/1
  d(Tp6_otsg)/dt/1 -> Tp6_otsg/1
  Tp6_otsg/1 -> [Tp6], Display30/1, HITEC OUTLET TEMPERATURE/1, Mux/12
  d(Tw1_otsg)/dt/1 -> Tw1_otsg/1
  d(Tw2_otsg)/dt/1 -> Tw2_otsg/1
  Tw3_otsg/1 -> [Tw3], Display27/1, Mux/15
  d(Tw3_otsg)/dt/1 -> Tw3_otsg/1
  d(Tw4_otsg)/dt/1 -> Tw4_otsg/1
  Tw4_otsg/1 -> [Tw4], Display26/1, Mux/16
  Tw5_otsg/1 -> [Tw5], Display25/1, Mux/17
  d(Tw5_otsg)/dt/1 -> Tw5_otsg/1
  d(Tw6_otsg)/dt/1 -> Tw6_otsg/1
  Tw6_otsg/1 -> [Tw6], Display24/1, Mux/18
  L_sc/1 -> [subcool_level], Display4/1, Mux/30
  L_s/1 -> Unit Delay1/1
  L_b/1 -> [boil_level], Display6/1, Mux/28
  P_sat/1 -> Display38/1, Mux/34
  Tsc2_otsg/1 -> [subcool_temp], Display20/1, Mux/23
  d(Tsc2_otsg)/dt/1 -> Tsc2_otsg/1
  Ts2_otsg/1 -> [stm_temp2], Display22/1, Mux/21
  rho_b/1 -> Unit Delay/1
  Unit Delay/1 -> Display19/1, Mux/24
  Mux/1 -> W_b/1, W_db/1, d_M_s/dt/1, T_sat/1, dP_sc/dt/1, dP_sat/dt/1, dP_s/dt/1, d(L_sc)/dt/1, d(L_b)/dt/1, d(L_s)/dt/1, L_s/1, rho_b/1, d(Tsc2_otsg)/dt/1, d(Ts2_otsg)/dt/1, d(Ts1_otsg)/dt/1, d(Tw6_otsg)/dt/1, d(Tw5_otsg)/dt/1, d(Tw4_otsg)/dt/1, d(Tw3_otsg)/dt/1, d(Tw2_otsg)/dt/1, d(Tw1_otsg)/dt/1, d(Tp6_otsg)/dt/1, d(Tp5_otsg)/dt/1, d(Tp4_otsg)/dt/1, d(Tp3_otsg)/dt/1, d(Tp2_otsg)/dt/1, d(Tp1_otsg)/dt/1, Fcn1/1, M_s_fac1/1, Unit Delay4/1
  d(Ts1_otsg)/dt/1 -> Display23/1, Mux/20, Ts1_otsg/1
  d(Ts2_otsg)/dt/1 -> Display21/1, Mux/22, Ts2_otsg/1
  dP_s/dt/1 -> Display16/1, Mux/31, P_s/1
  d(L_b)/dt/1 -> Display7/1, Mux/27, L_b/1
  d(L_s)/dt/1 -> Display17/1, Mux/26
  d(L_sc)/dt/1 -> Display5/1, Mux/29, L_sc/1
  dP_sat/dt/1 -> Mux/33, P_sat/1
  dP_sc/dt/1 -> Display13/1, Mux/35, P_sc/1
  Unit Delay1/1 -> [steam_level], Display18/1, Mux/25
  T_sat/1 -> [Sat_temp], Display12/1, Mux/37
  M_s_fac1/1 -> Unit Delay2/1
  d_M_s/dt/1 -> Display10/1, Mux/38, M_s/1
  W_db/1 -> [sc2bl], Display3/1, Mux/41
  W_b/1 -> [bl2sh], Display2/1, Mux/42
  Unit Delay4/1 -> To Workspace/1
  Tw1_otsg/1 -> [Tw1], Display29/1, Mux/13
  From Workspace1/1 -> Display1/1, To File2/1, PID Controller (2DOF)1/1
  Ts1_otsg/1 -> [stm_temp], STEAM TEMPERATURE/1, Mux/19, Display8/1
  POWER/1 -> PID Controller (2DOF)1/2, Display/1
  Tw2_otsg/1 -> [Tw2], Display28/1, Mux/14
  P_s/1 -> [stm_pressure], Display15/1, Mux/32, STEAM PRESSURE/1
  Unit Delay2/1 -> [flow_out], STEAM FLOW RATE/1, Mux/40, Display11/1
  P_sc/1 -> [sbcool_pressure], Display14/1, Mux/36
  FEEDWATER INLET TEMPERATURE/1 -> [fdw_temp], Display37/1, Mux/2
  PID Controller (2DOF)1/1 -> Multiply/1
  Fcn1/1 -> Unit Delay3/1
  Unit Delay3/1 -> Display9/1
  From/1 -> Add/1, Multiply3/1
  From1/1 -> Multiply2/1, Add/2
  From2/1 -> Add/3, Multiply1/1
  Add/1 -> Total Length/1
  " "/1 -> "Actual Length "/1
  Multiply3/1 -> Add1/3
  Multiply2/1 -> Add1/2
  Multiply1/1 -> Add1/1
  Add1/1 -> Total Mass/1
  From4/1 -> Subtract1/1, Subtract/1
  From3/1 -> Subtract3/2, Subtract/2
  Subtract/1 -> Integrator/1
  M_s/1 -> Mux/39, Display41/1
  From5/1 -> Subtract2/1, Subtract1/2
  Subtract1/1 -> Integrator1/1
  Integrator1/1 -> Add2/1, Subcooled/1
  From6/1 -> Subtract2/2, Subtract3/1
  Integrator2/1 -> Add2/2, Boiling/1
  Subtract2/1 -> Integrator2/1
  Integrator3/1 -> Add2/3, Superheated/1
  Subtract3/1 -> Integrator3/1
  Add2/1 -> Added Mass/1
  Integrator/1 -> Overall Mass/1
  From7/1 -> Fdw Enthalpy/1
  From8/1 -> Fdw Enthalpy/2
  Fdw Enthalpy/1 -> Subtract4/1
  From9/1 -> Add3/2
  Product/1 -> Subtract6/1, Display42/1, SC Power/1
  From10/1 -> Add3/1
  Add3/1 -> Multiply4/1
  From11/1 -> SC Enthalpy/2
  From12/1 -> SC Enthalpy/1
  SC Enthalpy/1 -> Subtract4/2, Subtract5/1
  Multiply4/1 -> Product/1
  Subtract4/1 -> Product/2
  Stm Enthalpy/1 -> Subtract5/2
  From13/1 -> Stm Enthalpy/1
  From14/1 -> Stm Enthalpy/2
  From16/1 -> Add4/1
  Add4/1 -> Multiply5/1
  Multiply5/1 -> Product1/2
  From15/1 -> Add4/2
  Subtract5/1 -> Product1/1
  Product1/1 -> Subtract6/2, SH Power/1, Display43/1
  Subtract6/1 -> Display44/1, Sum Power/1
  From17/1 -> Subtract7/1
  From23/1 -> Subtract7/2
  From18/1 -> Subtract8/1
  From24/1 -> Subtract8/2
  From19/1 -> Subtract9/1
  From25/1 -> Subtract9/2
  From26/1 -> Subtract10/2
  From20/1 -> Subtract10/1
  From21/1 -> Subtract11/1
  From27/1 -> Subtract11/2
  From22/1 -> Subtract12/1
  From28/1 -> Subtract12/2
  Subtract7/1 -> Fcn2/1
  Subtract8/1 -> Fcn3/1
  Subtract9/1 -> Fcn4/1
  Subtract10/1 -> Fcn5/1
  Subtract11/1 -> Fcn6/1
  Subtract12/1 -> Fcn7/1
  Fcn2/1 -> Display45/1, Add5/1
  Fcn3/1 -> Display46/1, Add5/2
  Fcn4/1 -> Display47/1, Add5/3
  Fcn5/1 -> Display48/1, Add5/4
  Fcn6/1 -> Display49/1, Add5/5
  Fcn7/1 -> Display50/1, Add5/6
  Add5/1 -> Htc2Wall/1
  Fcn9/1 -> Display52/1, Add6/2
  Add6/1 -> Wall2Sec/1
  Fcn10/1 -> Display53/1, Add6/3
  Fcn12/1 -> Display55/1, Add6/5
  Fcn13/1 -> Display56/1, Add6/6
  Fcn11/1 -> Display54/1, Add6/4
  Subtract16/1 -> Fcn8/1
  From36/1 -> Subtract17/1
  Fcn8/1 -> Display51/1, Add6/1
  Subtract13/1 -> Fcn11/1
  Subtract15/1 -> Fcn13/1
  From35/1 -> Subtract16/1
  Subtract17/1 -> Fcn9/1
  Subtract18/1 -> Fcn10/1
  Subtract14/1 -> Fcn12/1
  From40/1 -> Subtract15/1
  From39/1 -> Subtract14/1
  From37/1 -> Subtract18/1
  From38/1 -> Subtract13/1
  From29/1 -> Subtract14/2
  From30/1 -> Subtract13/2
  From31/1 -> Subtract18/2
  From32/1 -> Subtract16/2
  From33/1 -> Subtract17/2
  From34/1 -> Subtract15/2
  "Feedwater Flow "/1 -> ?
  Multiply/1 -> FdW Flow/1, Signal 5/1, [flow_in], Mux/5

== system Nerthus_sim/TEST BLOCKS/Primary loop constant heat production ==
  In1 : Inport
  Fcn : Fcn  Expr=u(1) + P/(vdot_f*rho_f*scp_f)
  Mux : Mux  Inputs=2
  Out1 : Outport  VectorParamsAs1DForOutWhenUnconnected=off
  wires:
  In1/1 -> Mux/1
  Fcn/1 -> Out1/1, Mux/2
  Mux/1 -> Fcn/1

== system Nerthus_sim/TEST BLOCKS/Primary loop constant heat removal ==
  In1 : Inport
  Fcn : Fcn  Expr=u(1) - P/(vdot_f*rho_f*scp_f)
  Mux : Mux  Inputs=2
  Out1 : Outport  VectorParamsAs1DForOutWhenUnconnected=off
  wires:
  In1/1 -> Mux/1
  Fcn/1 -> Out1/1, Mux/2
  Mux/1 -> Fcn/1

== system Nerthus_sim/TEST BLOCKS/Secondaary loop constant heat production ==
  In1 : Inport
  Fcn : Fcn  Expr=u(1) + P/(vdot_s*rho_s*scp_s)
  Mux : Mux  Inputs=2
  Out1 : Outport  VectorParamsAs1DForOutWhenUnconnected=off
  wires:
  In1/1 -> Mux/1
  Fcn/1 -> Out1/1, Mux/2
  Mux/1 -> Fcn/1
